simulink model "modified_major_project"  (Simulink 10.3)
settings: Solver=VariableStepAuto  StartTime=0.0  StopTime=1  RelTol=1e-3
libraries: spsMosfetLib x6, spsMeanLib x4, spsSeriesRLCBranchLib x4, spsCurrentMeasurementLib x3, spsDiodeLib x3, spsVoltageMeasurementLib x3, spspowerguiLib x2, spsIGBTDiodeLib x1, spsDCVoltageSourceLib x1, pid_lib x1, spsPermanentMagnetSynchronousMachineLib x1, simulink x1
settings Model: Creator=Edde Nikhil  LastModifiedBy=Edde Nikhil
settings SolverCC: AlgebraicLoopSolver=Auto
settings DataIOCC: SaveFormat=Dataset  SignalLoggingSaveFormat=Dataset  ReturnWorkspaceOutputs=on
settings OptimizationCC: ExpressionDepthLimit=128  LifeSpan=auto
settings DebuggingCC: UnderspecifiedInitializationDetection=Simplified  MergeDetectMultiDrivingBlocksExec=error  FcnCallInpInsideContextMsg=error  StateNameClashWarn=none  SFUnexpectedBacktrackingDiag=error  SFNoUnconditionalDefaultTransitionDiag=error  SFExecutionAtInitializationDiag=warning  SFMachineParentedDataDiag=error  ArithmeticOperatorsInVariantConditions=error
settings HardwareCC: ProdBitPerPointer=64  ProdBitPerSizeT=64  ProdBitPerPtrDiffT=64  ProdLargestAtomicFloat=Float  ProdIntDivRoundTo=Zero  ProdEndianess=LittleEndian  ProdWordSize=64  ProdHWDeviceType=Intel->x86-64 (Windows64)
settings ModelReferenceCC: PropagateSignalLabelsOutOfModel=on
settings SFSimCC: SimUseLocalCustomCode=on  CustomCodeUndefinedFunction=FilterOut
settings RTWCC: RTWUseLocalCustomCode=on
settings CodeAppCC: StateflowObjectComments=off
settings GRTTargetCC: TargetLangStandard=C99 (ISO)  CombineOutputUpdateFcns=on  GRTInterface=off
settings ConfigComp: CovMetricSettings=dwe  CovSaveCumulativeToWorkspaceVar=off  CovSaveSingleToWorkspaceVar=off  CovExternalEMLEnable=on

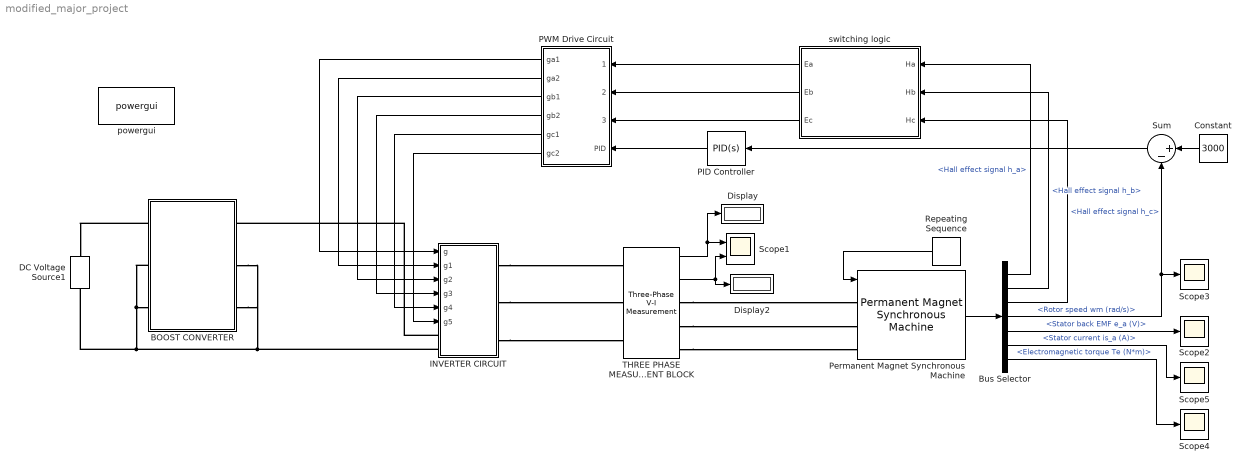
== system modified_major_project ==
  BOOST CONVERTER : Subsystem
  Bus Selector : BusSelector  OutputSignals=Hall effect signal h_a,Hall effect signal h_b,Hall effect signal h_c,Rotor speed wm (rad/s),Stator back EMF e_a (V),Stator current is_a (A),Electromagnetic torque Te (N*m)
  Constant : Constant  Value=3000  VectorParams1D=off  OutMax=[30000]  LockScale=on
  DC Voltage Source1 : spsDCVoltageSourceLib/DC Voltage Source  Amplitude=200  Measurements=None
  Display : Display
  Display2 : Display
  INVERTER CIRCUIT : Subsystem
  PID Controller : pid_lib/PID Controller  Controller=PID  Form=Parallel  TimeDomain=Continuous-time  UseExternalTs=off  SampleTime=-1  IntegratorMethod=Forward Euler  FilterMethod=Forward Euler  ControllerParametersSource=internal  P=1  I=1  D=0  UseFilter=on  N=100  TunerSelectOption=Transfer Function Based (PID Tuner App)  InitialConditionSource=internal  InitialConditionForIntegrator=0  InitialConditionForFilter=0  DifferentiatorICPrevScaledInput=0  ExternalReset=none  TrackingMode=off  Kt=1  LimitOutput=off  SatLimitsSource=internal  UpperSaturationLimit=inf  LowerSaturationLimit=-inf  LinearizeAsGain=on  AntiWindupMode=none  Kb=1  POutMin=[]  POutMax=[]  IOutMin=[]  IOutMax=[]  DOutMin=[]  DOutMax=[]  NOutMin=[]  NOutMax=[]  SumOutMin=[]  SumOutMax=[]  SaturationOutMin=[]  SaturationOutMax=[]  PParamMin=[]  PParamMax=[]  IParamMin=[]  IParamMax=[]  DParamMin=[]  DParamMax=[]  NParamMin=[]  NParamMax=[]  KbParamMin=[]  KbParamMax=[]  KtParamMin=[]  KtParamMax=[]  KbOutMin=[]  KbOutMax=[]  KtOutMin=[]  KtOutMax=[]  IntegratorOutMin=[]  IntegratorOutMax=[]  FilterOutMin=[]  FilterOutMax=[]  SumI1OutMin=[]  SumI1OutMax=[]  SumI2OutMin=[]  SumI2OutMax=[]  SumI3OutMin=[]  SumI3OutMax=[]  SumI4OutMin=[]  SumI4OutMax=[]  SumDOutMin=[]  SumDOutMax=[]  DifferentiatorOutMin=[]  DifferentiatorOutMax=[]  FilterDiffOutCoefMin=[]  FilterDiffOutCoefMax=[]  ReciprocalOutMin=[]  ReciprocalOutMax=[]  SumDenOutMin=[]  SumDenOutMax=[]  SumNumOutMin=[]  SumNumOutMax=[]  DivideOutMin=[]  DivideOutMax=[]  UdiffTsProdOutMin=[]  UdiffTsProdOutMax=[]  NTsProdOutMin=[]  NTsProdOutMax=[]  UintegralTsProdOutMin=[]  UintegralTsProdOutMax=[]  UngainTsProdOutMin=[]  UngainTsProdOutMax=[]  IntegratorContinuousStateAttributes=''  IntegratorStateMustResolveToSignalObject=off  IntegratorRTWStateStorageClass=Auto  FilterContinuousStateAttributes=''  FilterStateMustResolveToSignalObject=off  FilterRTWStateStorageClass=Auto  ParallelPVariant=InternalParameters  IdealPVariant=Disabled  IVariant=InternalParameters  DVariant=InternalParameters  IntegratorVariant=Continuous  SatVariant=Disabled  AWVariant=Passthrough  PCopyVariant=Disabled  TRVariant=Disabled  FdbkBlocksVariant=Forward  IdealPFdbkVariant=Disabled  SatFdbkVariant=Disabled  DerivativeFilterVariant=ContFilter  NVariant=InternalParameters  NCopyVariant=Disabled  FilterICVariant=InternalICsFilter  IntegratorICVariant=InternalICs  ExternalResetVariant=Disabled  TRSumVariant=Passthrough  SumFdbkVariant=Disabled  SumVariant=Sum_PID  TsampFilterVariant=InternalTs  TsampNgainVariant=Passthrough  TsampIntegralVariant=Passthrough  ExternalSaturationOutDataTypeStr=Inherit: Same as second input
  PWM Drive Circuit : Subsystem
  Permanent Magnet Synchronous Machine : spsPermanentMagnetSynchronousMachineLib/Permanent Magnet Synchronous Machine  NbPhases=3  FluxDistribution=Trapezoidal  RotorType=Round  MechanicalLoad=Torque Tm  PresetModel=No  ShowDetailedParameters=on  MeasurementBus=off  Resistance=3.58  Inductance=9.13e-3  dqInductances=[8.5e-3,8.5e-3]  La=0.000395  MachineConstant=Torque Constant (N.m / A_peak)  Flux=0.16234  VoltageCst=67.9998  TorqueCst=0.64935  Flat=120  Mechanical=[0.0027 0.0004924 2 0]  PolePairs=4  InitialConditions=[0,0, 0,0]  InitialConditions5ph=[0 0 0 0 0 0]  RefAngle=90 degrees behind phase A axis (modified Park)  IterativeDiscreteModel=Trapezoidal non iterative  TsBlock=-1  TsPowergui=0
  Repeating Sequence : simulink/Sources/Repeating Sequence  rep_seq_t=[0 1]  rep_seq_y=[0 1]
  Scope1 : Scope  NumInputPorts=2
  Scope{2..5} (4 alike) : Scope
  Sum : Sum  Inputs=|+-
  THREE PHASE MEASUREMENT BLOCK : spsThreePhaseVIMeasurementLib/Three-Phase V-I Measurement  VoltageMeasurement=phase-to-phase  SetLabelV=off  LabelV=Vabc  Vpu=off  VpuLL=off  CurrentMeasurement=yes  SetLabelI=off  LabelI=Iabc  Ipu=off  Pbase=100e6  Vbase=500e3  OutputType=Complex  PhasorSimulation=off  PSBequivalent=0
  powergui : spspowerguiLib/powergui  Priority=1  SimulationMode=Continuous  SampleTime=1e-7  frequency=60  Iterations=50  frequencyindice=0  Pbase=100e6  ErrMax=1e-4  UnitsV=kV  UnitsW=MW  buscounter=0  FunctionMessages=off  echomessages=off  EnableUseOfTLC=off  CurrentSourceSwitches=off  DisableSnubberDevices=off  DisableRonSwitches=off  DisableVfSwitches=off  DisplayEquations=off  AutomaticDiscreteSolvers=off  SolverType=Tustin/Backward Euler (TBE)  Interpol=off  ExternalGateDelay=off  methode=off  Ts=100  x0status=blocks  SPID=on  SwTol=0  HookPort=off  NonlinearTolerance=0  nMaxIteration=15  ContinueOnMaxIteration=off  RestoreLinks=warning  ResistiveCurrentMeasurement=off  Frange=[0:2:500]  Ylog=off  Xlog=on  ShowGrid=off  save=off  variable=ZData  structure=0  ZoomFFT=off  StartTime=0.0  cycles=1  DisplayStyle=1  fundamental=60  FreqAxis=off  MaxFrequency=1000  frequencyindicesteady=1  RmsSteady=1  display=off
  switching logic : Subsystem
  wires:
  switching logic/1(Ea) -> PWM Drive Circuit/1("1 ")
  switching logic/2(Eb) -> PWM Drive Circuit/2(2)
  Permanent Magnet Synchronous Machine/1 -> Bus Selector/1
  Bus Selector/1 -> switching logic/1(Ha)  "<Hall effect signal h_a>"
  Repeating Sequence/1 -> Permanent Magnet Synchronous Machine/1
  Sum/1 -> PID Controller/1
  PID Controller/1 -> PWM Drive Circuit/4(PID)
  Bus Selector/4 -> Sum/2, Scope3/1  "<Rotor speed wm (rad/s)>"
  Bus Selector/7 -> Scope4/1  "<Electromagnetic torque Te (N*m)>"
  Bus Selector/6 -> Scope5/1  "<Stator current is_a (A)>"
  Bus Selector/5 -> Scope2/1  "<Stator back EMF e_a (V)>"
  Bus Selector/3 -> switching logic/3(Hc)  "<Hall effect signal h_c>"
  switching logic/3(Ec) -> PWM Drive Circuit/3(3)
  Bus Selector/2 -> switching logic/2(Hb)  "<Hall effect signal h_b>"
  Constant/1 -> Sum/1
  THREE PHASE MEASUREMENT BLOCK/1 -> Display/1, Scope1/1
  THREE PHASE MEASUREMENT BLOCK/2 -> Display2/1, Scope1/2
  PWM Drive Circuit/1(ga1) -> INVERTER CIRCUIT/1(g)
  PWM Drive Circuit/2(ga2) -> INVERTER CIRCUIT/2(g1)
  PWM Drive Circuit/3(gb1) -> INVERTER CIRCUIT/3(g2)
  PWM Drive Circuit/4(gb2) -> INVERTER CIRCUIT/4(g3)
  PWM Drive Circuit/5(gc1) -> INVERTER CIRCUIT/5(g4)
  PWM Drive Circuit/6(gc2) -> INVERTER CIRCUIT/6(g5)
  connections:
  THREE PHASE MEASUREMENT BLOCK/RConn1 -- Permanent Magnet Synchronous Machine/LConn1
  THREE PHASE MEASUREMENT BLOCK/RConn3 -- Permanent Magnet Synchronous Machine/LConn3
  THREE PHASE MEASUREMENT BLOCK/RConn2 -- Permanent Magnet Synchronous Machine/LConn2
  BOOST CONVERTER/LConn2 -- BOOST CONVERTER/RConn3 -- BOOST CONVERTER/RConn2 -- INVERTER CIRCUIT/LConn2 -- DC Voltage Source1/LConn1 -- BOOST CONVERTER/LConn3
  BOOST CONVERTER/LConn1 -- DC Voltage Source1/RConn1
  INVERTER CIRCUIT/LConn1 -- BOOST CONVERTER/RConn1
  INVERTER CIRCUIT/RConn1 -- THREE PHASE MEASUREMENT BLOCK/LConn1
  INVERTER CIRCUIT/RConn2 -- THREE PHASE MEASUREMENT BLOCK/LConn2
  INVERTER CIRCUIT/RConn3 -- THREE PHASE MEASUREMENT BLOCK/LConn3

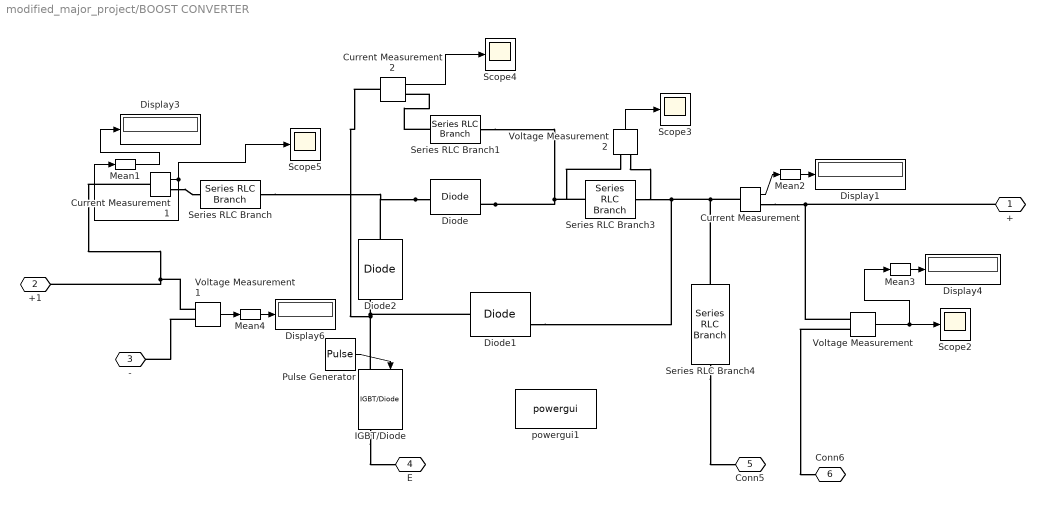
== system modified_major_project/BOOST CONVERTER ==
  Current Measurement : spsCurrentMeasurementLib/Current Measurement  PhasorSimulation=off  OutputType=Complex  PSBequivalent=0
  Current Measurement1 : spsCurrentMeasurementLib/Current Measurement  PhasorSimulation=off  OutputType=Complex  PSBequivalent=0
  Current Measurement2 : spsCurrentMeasurementLib/Current Measurement  PhasorSimulation=off  OutputType=Complex  PSBequivalent=0
  Diode : spsDiodeLib/Diode  Ron=0.001  Lon=0  Vf=0.8  IC=0  UseSnubber=0  Rs=50000  Cs=250e-9  Measurements=on
  Diode1 : spsDiodeLib/Diode  Ron=0.001  Lon=0  Vf=0.8  IC=0  UseSnubber=0  Rs=50000  Cs=250e-9  Measurements=on
  Diode2 : spsDiodeLib/Diode  Ron=0.001  Lon=0  Vf=0.8  IC=0  UseSnubber=0  Rs=50000  Cs=250e-9  Measurements=on
  Display{1,3..4,6} (4 alike) : Display
  IGBT/Diode : spsIGBTDiodeLib/IGBT//Diode  Ron=1e-3  Rs=1e5  Cs=inf  Measurements=on
  Mean{1..4} (4 alike) : spsMeanLib/Mean  Freq=60  Vinit=0  Ts=0
  Pulse Generator : DiscretePulseGenerator  PulseType=Time based  Period=1/50000  PulseWidth=13.9
  Scope{2..5} (4 alike) : Scope
  Series RLC Branch : spsSeriesRLCBranchLib/Series RLC Branch  LConnTagsString=__new0  RConnTagsString=__new0  BranchType=L  Resistance=1  Inductance=0.556e-3  SetiL0=off  InitialCurrent=0  Capacitance=1e-6  Setx0=off  InitialVoltage=0  Measurements=None
  Series RLC Branch1 : spsSeriesRLCBranchLib/Series RLC Branch  LConnTagsString=__new0  RConnTagsString=__new0  BranchType=L  Resistance=1  Inductance=0.6457e-3  SetiL0=off  InitialCurrent=0  Capacitance=1e-6  Setx0=off  InitialVoltage=0  Measurements=None
  Series RLC Branch3 : spsSeriesRLCBranchLib/Series RLC Branch  LConnTagsString=__new0  RConnTagsString=__new0  BranchType=C  Resistance=1  Inductance=1e-3  SetiL0=off  InitialCurrent=0  Capacitance=1.37e-6  Setx0=off  InitialVoltage=0  Measurements=None
  Series RLC Branch4 : spsSeriesRLCBranchLib/Series RLC Branch  LConnTagsString=__new0  RConnTagsString=__new0  BranchType=C  Resistance=1  Inductance=1e-3  SetiL0=off  InitialCurrent=0  Capacitance=300e-6  Setx0=off  InitialVoltage=0  Measurements=None
  Voltage Measurement : spsVoltageMeasurementLib/Voltage Measurement  PhasorSimulation=off  OutputType=Complex  PSBequivalent=0
  Voltage Measurement1 : spsVoltageMeasurementLib/Voltage Measurement  PhasorSimulation=off  OutputType=Complex  PSBequivalent=0
  Voltage Measurement2 : spsVoltageMeasurementLib/Voltage Measurement  PhasorSimulation=off  OutputType=Complex  PSBequivalent=0
  powergui1 : spspowerguiLib/powergui  Priority=1  SimulationMode=Discrete  SampleTime=1e-7  frequency=60  Iterations=50  frequencyindice=0  Pbase=100e6  ErrMax=1e-4  UnitsV=kV  UnitsW=MW  buscounter=0  FunctionMessages=off  echomessages=off  EnableUseOfTLC=off  CurrentSourceSwitches=off  DisableSnubberDevices=off  DisableRonSwitches=off  DisableVfSwitches=off  DisplayEquations=off  AutomaticDiscreteSolvers=off  SolverType=Tustin/Backward Euler (TBE)  Interpol=off  ExternalGateDelay=off  methode=off  Ts=100  x0status=blocks  SPID=on  SwTol=0  HookPort=off  NonlinearTolerance=1e-4  nMaxIteration=100  ContinueOnMaxIteration=off  RestoreLinks=warning  ResistiveCurrentMeasurement=off  Frange=[0:2:500]  Ylog=off  Xlog=on  ShowGrid=off  save=off  variable=ZData  structure=0  ZoomFFT=off  StartTime=0.0  cycles=1  DisplayStyle=1  fundamental=60  FreqAxis=off  MaxFrequency=1000  frequencyindicesteady=1  RmsSteady=1  display=off
  + : PMIOPort  Side=Right
  +1 : PMIOPort  Port=2  Side=Left
  - : PMIOPort  Port=3  Side=Left
  E : PMIOPort  Port=4  Side=Right
  Conn5 : PMIOPort  Port=5  Side=Right
  Conn6 : PMIOPort  Port=6  Side=Left
  wires:
  Pulse Generator/1 -> IGBT/Diode/1
  Mean4/1 -> Display6/1
  Mean3/1 -> Display4/1
  Current Measurement2/1 -> Scope4/1
  Voltage Measurement1/1 -> Mean4/1
  Current Measurement1/1 -> Mean1/1, Scope5/1
  Mean1/1 -> Display3/1
  Voltage Measurement/1 -> Mean3/1, Scope2/1
  Mean2/1 -> Display1/1
  Current Measurement/1 -> Mean2/1
  Voltage Measurement2/1 -> Scope3/1
  connections:
  Diode/RConn1 -- Series RLC Branch1/RConn1 -- Series RLC Branch3/LConn1 -- Voltage Measurement2/LConn1
  Diode2/RConn1 -- Diode1/LConn1 -- Current Measurement2/LConn1 -- IGBT/Diode/LConn1
  Current Measurement1/LConn1 -- +1/RConn1 -- Voltage Measurement1/LConn1
  Voltage Measurement/LConn2 -- Conn6/RConn1
  Current Measurement/RConn1 -- Voltage Measurement/LConn1 -- +/RConn1
  Voltage Measurement1/LConn2 -- -/RConn1
  Current Measurement1/RConn1 -- Series RLC Branch/LConn1
  Series RLC Branch4/LConn1 -- Series RLC Branch3/RConn1 -- Voltage Measurement2/LConn2 -- Diode1/RConn1 -- Current Measurement/LConn1
  Diode/LConn1 -- Series RLC Branch/RConn1 -- Diode2/LConn1
  Series RLC Branch1/LConn1 -- Current Measurement2/RConn1
  Series RLC Branch4/RConn1 -- Conn5/RConn1
  IGBT/Diode/RConn1 -- E/RConn1

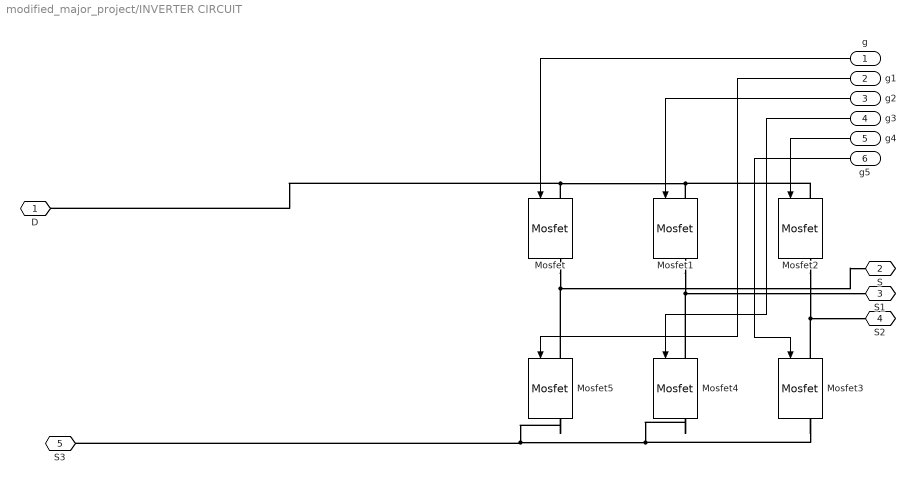
== system modified_major_project/INVERTER CIRCUIT ==
  g : Inport
  g1 : Inport  Port=2
  g2 : Inport  Port=3
  g3 : Inport  Port=4
  g4 : Inport  Port=5
  g5 : Inport  Port=6
  Mosfet{,1..5} (6 alike) : spsMosfetLib/Mosfet  Ron=0.1  Lon=0  Rd=0.01  Vfd=0  IC=0  Rs=1e5  Cs=inf  Measurements=on
  D : PMIOPort  Side=Left
  S : PMIOPort  Port=2  Side=Right
  S1 : PMIOPort  Port=3  Side=Right
  S2 : PMIOPort  Port=4  Side=Right
  S3 : PMIOPort  Port=5  Side=Left
  wires:
  g1/1 -> Mosfet5/1
  g5/1 -> Mosfet3/1
  g3/1 -> Mosfet4/1
  g4/1 -> Mosfet2/1
  g/1 -> Mosfet/1
  g2/1 -> Mosfet1/1
  connections:
  Mosfet3/LConn1 -- S2/RConn1 -- Mosfet2/RConn1
  Mosfet/LConn1 -- D/RConn1 -- Mosfet2/LConn1 -- Mosfet1/LConn1
  Mosfet4/LConn1 -- S1/RConn1 -- Mosfet1/RConn1
  Mosfet5/LConn1 -- Mosfet/RConn1 -- S/RConn1
  Mosfet4/RConn1 -- Mosfet3/RConn1 -- S3/RConn1 -- Mosfet5/RConn1

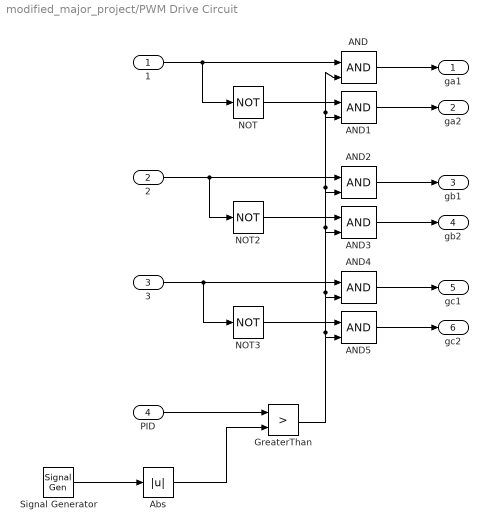
== system modified_major_project/PWM Drive Circuit ==
  "1 " : Inport
  2 : Inport  Port=2
  3 : Inport  Port=3
  PID : Inport  Port=4
  AND{,1..5} (6 alike) : Logic  IconShape=distinctive  AllPortsSameDT=off  OutDataTypeStr=boolean
  Abs : Abs
  GreaterThan : RelationalOperator  Operator=>  OutDataTypeStr=boolean  RndMeth=Simplest
  NOT : Logic  Operator=NOT  IconShape=distinctive  AllPortsSameDT=off  OutDataTypeStr=boolean
  NOT2 : Logic  Operator=NOT  IconShape=distinctive  AllPortsSameDT=off  OutDataTypeStr=boolean
  NOT3 : Logic  Operator=NOT  IconShape=distinctive  AllPortsSameDT=off  OutDataTypeStr=boolean
  Signal Generator : SignalGenerator  VectorParams1D=off
  ga1 : Outport  VectorParamsAs1DForOutWhenUnconnected=off
  ga2 : Outport  Port=2  VectorParamsAs1DForOutWhenUnconnected=off
  gb1 : Outport  Port=3  VectorParamsAs1DForOutWhenUnconnected=off
  gb2 : Outport  Port=4  VectorParamsAs1DForOutWhenUnconnected=off
  gc1 : Outport  Port=5  VectorParamsAs1DForOutWhenUnconnected=off
  gc2 : Outport  Port=6  VectorParamsAs1DForOutWhenUnconnected=off
  wires:
  AND/1 -> ga1/1
  AND1/1 -> ga2/1
  AND2/1 -> gb1/1
  AND3/1 -> gb2/1
  AND4/1 -> gc1/1
  AND5/1 -> gc2/1
  GreaterThan/1 -> AND5/2, AND4/2, AND3/2, AND2/2, AND1/2, AND/2
  "1 "/1 -> NOT/1, AND/1
  NOT/1 -> AND1/1
  NOT2/1 -> AND3/1
  NOT3/1 -> AND5/1
  2/1 -> NOT2/1, AND2/1
  3/1 -> NOT3/1, AND4/1
  PID/1 -> GreaterThan/1
  Abs/1 -> GreaterThan/2
  Signal Generator/1 -> Abs/1

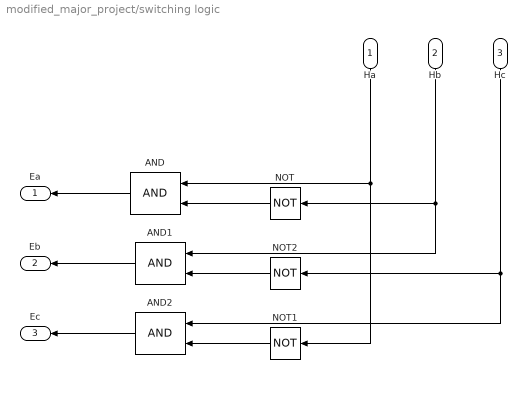
== system modified_major_project/switching logic ==
  Ha : Inport
  Hb : Inport  Port=2
  Hc : Inport  Port=3
  AND : Logic  IconShape=distinctive  AllPortsSameDT=off  OutDataTypeStr=boolean
  AND1 : Logic  IconShape=distinctive  AllPortsSameDT=off  OutDataTypeStr=boolean
  AND2 : Logic  IconShape=distinctive  AllPortsSameDT=off  OutDataTypeStr=boolean
  NOT : Logic  Operator=NOT  IconShape=distinctive  AllPortsSameDT=off  OutDataTypeStr=boolean
  NOT1 : Logic  Operator=NOT  IconShape=distinctive  AllPortsSameDT=off  OutDataTypeStr=boolean
  NOT2 : Logic  Operator=NOT  IconShape=distinctive  AllPortsSameDT=off  OutDataTypeStr=boolean
  Ea : Outport  VectorParamsAs1DForOutWhenUnconnected=off
  Eb : Outport  Port=2  VectorParamsAs1DForOutWhenUnconnected=off
  Ec : Outport  Port=3  VectorParamsAs1DForOutWhenUnconnected=off
  wires:
  Ha/1 -> NOT1/1, AND/1
  Hb/1 -> NOT/1, AND1/1
  Hc/1 -> AND2/1, NOT2/1
  NOT/1 -> AND/2
  NOT2/1 -> AND1/2
  NOT1/1 -> AND2/2
  AND/1 -> Ea/1
  AND1/1 -> Eb/1
  AND2/1 -> Ec/1
